simulink model "Simulink_v1"  (R2024b)
settings: Solver=FixedStepDiscrete  StartTime=0.0  StopTime=10.0  RelTol=1e-3
undefined symbols (not defined in the file or in its folder): DiscIntNeverNeededParam, ref
libraries: simulink x1
settings Model: Creator=johan  LastModifiedBy=johan
settings OptimizationCC: DefaultParameterBehavior=Inlined  GainParamInheritBuiltInType=on  UseFloatMulNetSlope=on  InlineInvariantSignals=on  ZeroExternalMemoryAtStartup=off  ZeroInternalMemoryAtStartup=off  EfficientFloat2IntCast=on
settings SFSimCC: SimTargetLang=C++
settings RTWCC: RTWVerbose=off  BuildConfiguration=Faster Runs  TargetLang=C++
settings CodeAppCC: ForceParamTrailComments=on  MATLABSourceComments=on
settings GRTTargetCC: TargetLangStandard=C++11 (ISO)  MatFileLogging=off  CodeInterfacePackaging=C++ class  SupportNonFinite=off

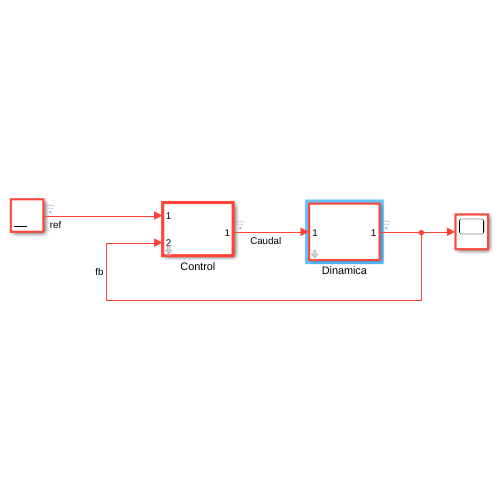
[thumbnail: Simulink's stored preview of the top-level diagram]
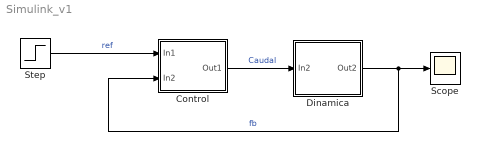
== system Simulink_v1 ==
  Control : Subsystem  TreatAsAtomicUnit=on  mask{Ts=1/1000, ki=5, kp=27}
      mask prompts: Ts "Sampling Time (Ts):"; ki "Integral (ki):"; kp "Proportional (kp):"
      mask DialogControl PI Prompt: Valores del controlador
  Dinamica : Subsystem  mask{Ts=1/1000}
      mask prompts: Ts "Sampling Time (Ts):"
  Scope : Scope
  Step : Step  After=ref  SampleTime=1/1000
  wires:
  Control/1(Out1) -> Dinamica/1(In2)  "Caudal"
  Dinamica/1(Out2) -> Scope/1, Control/2(In2)  "fb"
  Step/1 -> Control/1(In1)  "ref"

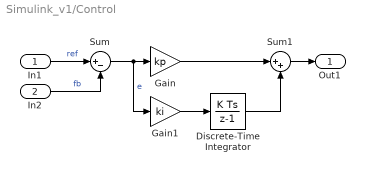
== system Simulink_v1/Control ==
  In1 : Inport
  In2 : Inport  Port=2
  Discrete-Time Integrator : DiscreteIntegrator  SampleTime=Ts  ICPrevOutput=DiscIntNeverNeededParam  ICPrevScaledInput=DiscIntNeverNeededParam
  Gain : Gain  Gain=kp
  Gain1 : Gain  Gain=ki
  Sum : Sum  Inputs=|+-
  Sum1 : Sum  Inputs=|++
  Out1 : Outport
  wires:
  In1/1 -> Sum/1  "ref"
  Sum/1 -> Gain1/1, Gain/1  "e"
  In2/1 -> Sum/2  "fb"
  Gain1/1 -> Discrete-Time Integrator/1
  Gain/1 -> Sum1/1
  Sum1/1 -> Out1/1
  Discrete-Time Integrator/1 -> Sum1/2

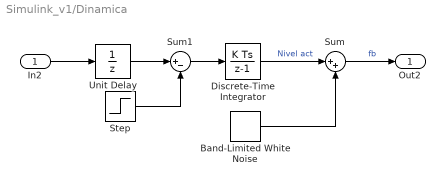
== system Simulink_v1/Dinamica ==
  In2 : Inport
  Band-Limited White Noise : simulink/Sources/Band-Limited White Noise  Cov=[0.000001]  Ts=Ts  seed=[23341]
  Discrete-Time Integrator : DiscreteIntegrator  SampleTime=Ts  ICPrevOutput=DiscIntNeverNeededParam  ICPrevScaledInput=DiscIntNeverNeededParam
  Step : Step  Time=3  After=5  SampleTime=Ts
  Sum : Sum  Inputs=|++
  Sum1 : Sum  Inputs=|+-
  Unit Delay : UnitDelay  SampleTime=Ts  HasFrameUpgradeWarning=on
  Out2 : Outport
  wires:
  In2/1 -> Unit Delay/1
  Discrete-Time Integrator/1 -> Sum/1  "Nivel act"
  Sum/1 -> Out2/1  "fb"
  Unit Delay/1 -> Sum1/1
  Sum1/1 -> Discrete-Time Integrator/1
  Step/1 -> Sum1/2
  Band-Limited White Noise/1 -> Sum/2
